simulink model "circuit_Rasp copia"  (R2018a)
settings: Solver=VariableStepAuto  StartTime=0.0  StopTime=10.0  RelTol=1e-3
libraries: pe_lib x10, fl_lib x6
settings Model: Creator=giovannirenda  LastModifiedBy=giovannirenda

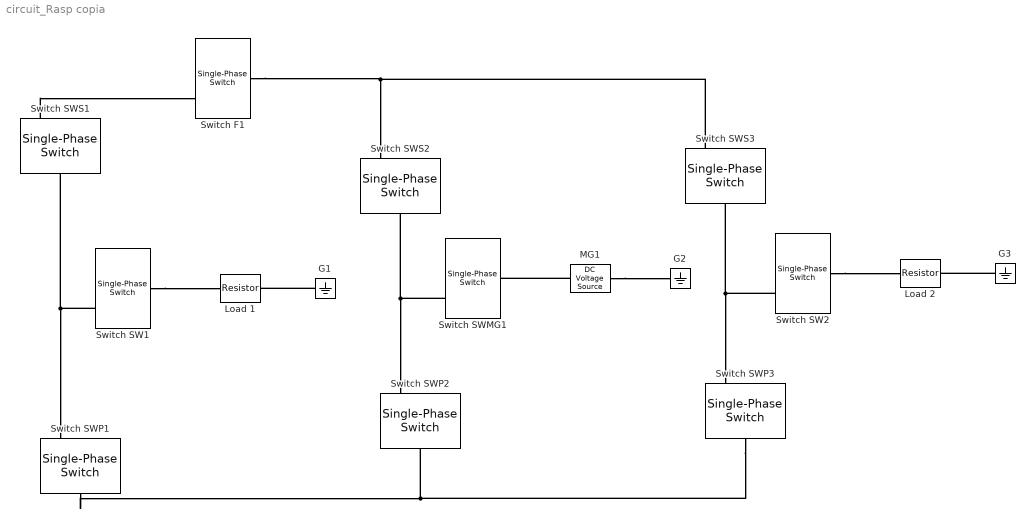
== system circuit_Rasp copia ==
  G1 : fl_lib/Electrical/Electrical Elements/Electrical Reference
  G2 : fl_lib/Electrical/Electrical Elements/Electrical Reference
  G3 : fl_lib/Electrical/Electrical Elements/Electrical Reference
  Load 1 : fl_lib/Electrical/Electrical Elements/Resistor  R=50 Ohm  i_specify=off  i_priority=None  i=0 A  i_nominal_specify=off  i_nominal_unit=A  i_nominal_value=1  v_specify=off  v_priority=None  v=0 V  v_nominal_specify=off  v_nominal_unit=V  v_nominal_value=1
  Load 2 : fl_lib/Electrical/Electrical Elements/Resistor  R=50 Ohm  i_specify=off  i_priority=None  i=0 A  i_nominal_specify=off  i_nominal_unit=A  i_nominal_value=1  v_specify=off  v_priority=None  v=0 V  v_nominal_specify=off  v_nominal_unit=V  v_nominal_value=1
  MG1 : fl_lib/Electrical/Electrical Sources/DC Voltage Source  v0=5000 V
  Switch F1 : pe_lib/Switches & Breakers/Fundamental Components/Single-Phase Switch  R_closed=0.001 Ohm  G_open=1e-6 1/Ohm  threshold=0 V
      settings: SourceProductName=Simscape Power Systems  SourceProductBaseCode=PS
  Switch SW1 : pe_lib/Switches & Breakers/Fundamental Components/Single-Phase Switch  R_closed=0.001 Ohm  G_open=1e-6 1/Ohm  threshold=0 V
      settings: SourceProductName=Simscape Power Systems  SourceProductBaseCode=PS
  Switch SW2 : pe_lib/Switches & Breakers/Fundamental Components/Single-Phase Switch  R_closed=0.001 Ohm  G_open=1e-6 1/Ohm  threshold=0 V
      settings: SourceProductName=Simscape Power Systems  SourceProductBaseCode=PS
  Switch SWMG1 : pe_lib/Switches & Breakers/Fundamental Components/Single-Phase Switch  R_closed=0.001 Ohm  G_open=1e-6 1/Ohm  threshold=0 V
      settings: SourceProductName=Simscape Power Systems  SourceProductBaseCode=PS
  Switch SWP1 : pe_lib/Switches & Breakers/Fundamental Components/Single-Phase Switch  R_closed=0.001 Ohm  G_open=1e-6 1/Ohm  threshold=0 V
      settings: SourceProductName=Simscape Power Systems  SourceProductBaseCode=PS
  Switch SWP2 : pe_lib/Switches & Breakers/Fundamental Components/Single-Phase Switch  R_closed=0.001 Ohm  G_open=1e-6 1/Ohm  threshold=0 V
      settings: SourceProductName=Simscape Power Systems  SourceProductBaseCode=PS
  Switch SWP3 : pe_lib/Switches & Breakers/Fundamental Components/Single-Phase Switch  R_closed=0.001 Ohm  G_open=1e-6 1/Ohm  threshold=0 V
      settings: SourceProductName=Simscape Power Systems  SourceProductBaseCode=PS
  Switch SWS1 : pe_lib/Switches & Breakers/Fundamental Components/Single-Phase Switch  R_closed=0.001 Ohm  G_open=1e-6 1/Ohm  threshold=0 V
      settings: SourceProductName=Simscape Power Systems  SourceProductBaseCode=PS
  Switch SWS2 : pe_lib/Switches & Breakers/Fundamental Components/Single-Phase Switch  R_closed=0.001 Ohm  G_open=1e-6 1/Ohm  threshold=0 V
      settings: SourceProductName=Simscape Power Systems  SourceProductBaseCode=PS
  Switch SWS3 : pe_lib/Switches & Breakers/Fundamental Components/Single-Phase Switch  R_closed=0.001 Ohm  G_open=1e-6 1/Ohm  threshold=0 V
      settings: SourceProductName=Simscape Power Systems  SourceProductBaseCode=PS
  connections:
  Switch SW1/LConn2 -- Switch SWP1/LConn2 -- Switch SWS1/RConn1
  Switch SW1/RConn1 -- Load 1/LConn1
  G1/LConn1 -- Load 1/RConn1
  Switch SWMG1/LConn2 -- Switch SWP2/LConn2 -- Switch SWS2/RConn1
  MG1/RConn1 -- G2/LConn1
  MG1/LConn1 -- Switch SWMG1/RConn1
  Switch SW2/LConn2 -- Switch SWS3/RConn1 -- Switch SWP3/LConn2
  Switch SW2/RConn1 -- Load 2/LConn1
  G3/LConn1 -- Load 2/RConn1
  Switch SWS3/LConn2 -- Switch F1/RConn1 -- Switch SWS2/LConn2
  Switch SWP1/RConn1 -- Switch SWP3/RConn1 -- Switch SWP2/RConn1
  Switch SWS1/LConn2 -- Switch F1/LConn2
